simulink model "BaseEngineController_LS"  (Simulink 7.7)
settings: Solver=FixedStepDiscrete  StartTime=0.0  StopTime=10.0  RelTol=1e-3
PreLoadFcn:
  | try, eval([bdroot '_setup']); catch, eval('model_setup', ''); end
InitFcn:
  | try, eval([bdroot '_setup']); catch, eval('model_setup', ''); end
undefined symbols (not defined in the file): ECU555, High, motohawk_build_version, motohawk_trunc_name, motohawk_vardec_config_group, motohawk_vardec_path, True
libraries: MotoHawk_lib x1418, motohawk_control_primitives_lib x183, motohawk_engine_lib x32, simulink x21, motohawk_annotations_lib x9, AutoDoc_lib x8, simulink_extras x4, motohawk_ccp_examples_lib x1, motohawk_control_primitives_motoshare_lib x1
(part 22 of 27)

== system BaseEngineController_LS/Foreground/Control/Controller/Run/MinGovernor/Idle State Determination ==
  Sensors : Inport
  MinGovOutput : Inport  Port=2
  TargetRPM : Inport  Port=3
  Bus Selector1 : BusSelector  OutputSignals=Raw.RPMInst
  Bus Selector2 : BusSelector  OutputSignals=RawProcessed.APPPcnt,RawProcessed.TPS
  Bus Selector3 : BusSelector  OutputSignals=RawProcessed.ETCRequest
  Constant : Constant  Value=true
  Data Type Conversion : DataTypeConversion  OutDataTypeStr=int16
  Determine if RPM is Falling : Subsystem
  IdleStateMachine : Stateflow chart  TreatAsAtomicUnit=on
      settings: RTWSystemCode=Function  RTWFcnNameOpts=Use subsystem name  RTWFileNameOpts=Use function name
  Logical Operator : Logic  OutDataTypeStr=boolean
  Multiport Switch : MultiPortSwitch  DataPortOrder=Zero-based contiguous  Inputs=2  zeroidx=on
  Multiport Switch1 : MultiPortSwitch  DataPortOrder=Zero-based contiguous  Inputs=2  zeroidx=on
  OnIdle State : motohawk_control_primitives_lib/CompareTo  SystemSampleTime=-1  op===  val=2
  Relational Operator : RelationalOperator  Operator=<  ZeroCross=off  InputSameDT=on
  Relational Operator1 : RelationalOperator  Operator=<  ZeroCross=off  InputSameDT=on
  Relational Operator2 : RelationalOperator  ZeroCross=off  InputSameDT=on
  Relational Operator3 : RelationalOperator  Operator=<  ZeroCross=off  InputSameDT=on
  Relational Operator4 : RelationalOperator  Operator=>  OutDataTypeStr=boolean
  Relational Operator5 : RelationalOperator  Operator=>  ZeroCross=off  InputSameDT=on
  Sum : Sum  Inputs=|++  SaturateOnIntegerOverflow=on  InputSameDT=on
  Sum1 : Sum  Inputs=++|  SaturateOnIntegerOverflow=on  InputSameDT=on
  Sum2 : Sum  Inputs=+-|  SaturateOnIntegerOverflow=on  InputSameDT=on
  Time Since Enabled (With Input)1 : motohawk_control_primitives_lib/Time Since Enabled (With Input)1  SystemSampleTime=-1  nam='IdleEnterTimer'  samp_time=.005  init=0  upperlim=16000
  motohawk_calibration1 : MotoHawk_lib/Calibration & Probing Blocks/motohawk_calibration  nam='EnableRPMFalling'  val=1  storage=Calibration  show_more=on  name_source=Use Parameter  data_type=Inherit via back propagation  read_level=1  write_level=1  ovr_cals=on  view_as=Number  enum_struct={'Disabled', 'Enabled'}  vector_style=Wide Row  use_help_units=on  help='If disabled, Min Gov will enable immediately after cranking without waiting for falling RPM.'  units='bool'  use_header_enum=off  row_header_enum={}  col_header_enum={}  use_min_max=on  min_val=0  max_val=1  use_precision=off  precision=''  gain=1  offset=0  exp=1  use_mototune_group=on  mototune_group=motohawk_vardec_path(gcb)
  motohawk_calibration2 : MotoHawk_lib/Calibration & Probing Blocks/motohawk_calibration  nam='MinGovEntryAirTimeThresh'  val=10  storage=Calibration  show_more=on  name_source=Use Parameter  data_type=Inherit from 'Default Value'  read_level=1  write_level=1  ovr_cals=on  view_as=Number  enum_struct={'Disabled', 'Enabled'}  vector_style=Wide Row  use_help_units=on  help='If entry AirPcnt condition is satisfied, but RPM is high, Min Gov will enable if this time is exceeded.'  units='s'  use_header_enum=off  row_header_enum={}  col_header_enum={}  use_min_max=on  min_val=-inf  max_val=inf  use_precision=off  precision=''  gain=1  offset=0  exp=1  use_mototune_group=on  mototune_group=motohawk_vardec_path(gcb)
  motohawk_calibration3 : MotoHawk_lib/Calibration & Probing Blocks/motohawk_calibration  nam='MinGovAirPcntHyst'  val=0.5  storage=Calibration  show_more=on  name_source=Use Parameter  data_type=Inherit from 'Default Value'  read_level=1  write_level=1  ovr_cals=on  view_as=Number  enum_struct={'Disabled', 'Enabled'}  vector_style=Wide Row  use_help_units=on  help='Hysteresis around MinGovEntryAirPcnt where Min Gov will disable.'  units='%'  use_header_enum=off  row_header_enum={}  col_header_enum={}  use_min_max=on  min_val=-inf  max_val=inf  use_precision=off  precision=''  gain=1  offset=0  exp=1  use_mototune_group=on  mototune_group=motohawk_vardec_path(gcb)
  motohawk_calibration4 : MotoHawk_lib/Calibration & Probing Blocks/motohawk_calibration  nam='InGearMinGovEntryRPMDelta'  val=75  storage=Calibration  show_more=on  name_source=Use Parameter  data_type=int16  read_level=1  write_level=1  ovr_cals=on  view_as=Number  enum_struct={'Disabled', 'Enabled'}  vector_style=Wide Row  use_help_units=on  help='RPM above setpoint where Min Gov will enable when RPM is falling into idle.'  units='RPM'  use_header_enum=off  row_header_enum={}  col_header_enum={}  use_min_max=on  min_val=-inf  max_val=inf  use_precision=off  precision=''  gain=1  offset=0  exp=1  use_mototune_group=on  mototune_group=motohawk_vardec_path(gcb)
  motohawk_calibration5 : MotoHawk_lib/Calibration & Probing Blocks/motohawk_calibration  nam='MinGovEntryAirPcnt'  val=3  storage=Calibration  show_more=on  name_source=Use Parameter  data_type=Inherit from 'Default Value'  read_level=1  write_level=1  ovr_cals=on  view_as=Number  enum_struct={'Disabled', 'Enabled'}  vector_style=Wide Row  use_help_units=on  help='Percent air (TPS or APP) position where below which Min Gov will enable.'  units='%'  use_header_enum=off  row_header_enum={}  col_header_enum={}  use_min_max=on  min_val=-inf  max_val=inf  use_precision=off  precision=''  gain=1  offset=0  exp=1  use_mototune_group=on  mototune_group=motohawk_vardec_path(gcb)
  motohawk_calibration6 : MotoHawk_lib/Calibration & Probing Blocks/motohawk_calibration  nam='StallSaverDeltaRPM'  val=10  storage=Calibration  show_more=on  name_source=Use Parameter  data_type=int16  read_level=1  write_level=1  ovr_cals=on  view_as=Number  enum_struct={'Disabled', 'Enabled'}  vector_style=Wide Row  use_help_units=on  help='RPM delta below setpoint where Min Gov will enable to prevent engine stalls.'  units='RPM'  use_header_enum=off  row_header_enum={}  col_header_enum={}  use_min_max=on  min_val=-inf  max_val=inf  use_precision=on  precision=''  gain=1  offset=0  exp=1  use_mototune_group=on  mototune_group=motohawk_vardec_path(gcb)
  motohawk_data_read1 : MotoHawk_lib/Data Storage Blocks/motohawk_data_read  source=Lookup By Name  structure=Scalar  operation=Read scalar from location by index  sz_vec=4  sz_row=2  sz_col=3  typ=boolean  nam='AirControlSource'  checkNull=on  struct_inst_name='Struct1'  struct_nam='MyStruct'
  motohawk_probe : MotoHawk_lib/Calibration & Probing Blocks/motohawk_probe  nam='RPMCtrlMode'  show_more=on  name_source=Use Parameter  read_level=1  view_as=Number  enum_struct={'Disabled', 'Enabled'}  vector_style=Wide Row  use_help_units=on  help=''  units=''  use_header_enum=off  row_header_enum={}  col_header_enum={}  use_precision=on  precision=''  gain=1  offset=0  exp=1  use_mototune_group=on  mototune_group=motohawk_vardec_path(gcb)
  motohawk_probe1 : MotoHawk_lib/Calibration & Probing Blocks/motohawk_probe  nam='IdleState'  show_more=on  name_source=Use Parameter  read_level=1  view_as=Enumeration  enum_struct={'Unknown', 'Flaring', 'OnIdle', 'OffIdle'}  vector_style=Wide Row  use_help_units=on  help='The idle governor may be one of: Flaring, OnIdle, OffIdle'  units=''  use_header_enum=off  row_header_enum={}  col_header_enum={}  use_precision=off  precision=''  gain=1  offset=0  exp=1  use_mototune_group=on  mototune_group=motohawk_vardec_path(gcb)
  OnIdle : Outport
  wires:
  Relational Operator3/1 -> IdleStateMachine/4(RPMLow)
  Sum2/1 -> Relational Operator3/2
  motohawk_calibration6/1 -> Sum2/2
  Relational Operator1/1 -> Time Since Enabled (With Input)1/1, IdleStateMachine/5(ThrCmdLow)
  Relational Operator/1 -> IdleStateMachine/3(RPMInRange)
  OnIdle State/1 -> OnIdle/1, motohawk_probe/1
  IdleStateMachine/1(IdleState) -> OnIdle State/1, motohawk_probe1/1
  motohawk_calibration5/1 -> Relational Operator1/2, Sum1/1
  Sum/1 -> Relational Operator/2
  motohawk_calibration4/1 -> Sum/1
  TargetRPM/1 -> Sum2/1, Sum/2
  Determine if RPM is Falling/1(RPM Falling) -> IdleStateMachine/2(RPMFalling)
  Sensors/1 -> Bus Selector1/1, Bus Selector2/1, Bus Selector3/1
  motohawk_calibration3/1 -> Sum1/2
  Sum1/1 -> Relational Operator2/2
  Bus Selector1/1 -> Determine if RPM is Falling/1(RPM), Data Type Conversion/1  "<RPMInst>"
  MinGovOutput/1 -> Relational Operator4/2
  Logical Operator/1 -> IdleStateMachine/6(ThrCmdHigh)
  Relational Operator2/1 -> Logical Operator/1
  motohawk_calibration1/1 -> IdleStateMachine/1(IdleEnable)
  Time Since Enabled (With Input)1/1 -> Relational Operator5/1
  motohawk_calibration2/1 -> Relational Operator5/2
  Relational Operator5/1 -> IdleStateMachine/7(APPTimeThresh)
  Multiport Switch1/1 -> Relational Operator1/1, Relational Operator2/1
  Bus Selector2/1 -> Multiport Switch1/2  "<APPPcnt>"
  Bus Selector2/2 -> Multiport Switch1/3  "<TPS>"
  motohawk_data_read1/1 -> Multiport Switch1/1, Multiport Switch/1
  Bus Selector3/1 -> Relational Operator4/1  "<ETCRequest>"
  Multiport Switch/1 -> Logical Operator/2
  Relational Operator4/1 -> Multiport Switch/2
  Constant/1 -> Multiport Switch/3
  Data Type Conversion/1 -> Relational Operator3/1, Relational Operator/1

== system BaseEngineController_LS/Foreground/Control/Controller/Run/MinGovernor/MotoringDetection ==
  ActualRPM : Inport
  SetpointRPM : Inport  Port=2
  Data Type Conversion : DataTypeConversion  SaturateOnIntegerOverflow=on  RndMeth=Zero
  Relational Operator1 : RelationalOperator  Operator=>
  Relational Operator2 : RelationalOperator  Operator=>
  Sum : Sum  Inputs=+-  SaturateOnIntegerOverflow=on
  Time Since Enabled (With Input)2 : motohawk_control_primitives_lib/Time Since Enabled (With Input)1  SystemSampleTime=-1  nam='MotoringTimer'  samp_time=.005  init=0  upperlim=16000
  motohawk_calibration1 : MotoHawk_lib/Calibration & Probing Blocks/motohawk_calibration  nam='MotoringDtctTimerLimit'  val=5  storage=Calibration  show_more=on  name_source=Use Parameter  data_type=Inherit from 'Default Value'  read_level=1  write_level=1  ovr_cals=on  view_as=Number  enum_struct={'Disabled', 'Enabled'}  vector_style=Wide Row  use_help_units=on  help='Amount of time engine speed has to be above the min gov. rpm set pt to set motoring flag.'  units='sec'  use_header_enum=off  row_header_enum={}  col_header_enum={}  use_min_max=off  min_val=0  max_val=100  use_precision=off  precision=''  gain=1  offset=0  exp=1  use_mototune_group=on  mototune_group=motohawk_vardec_path(gcb)
  motohawk_calibration3 : MotoHawk_lib/Calibration & Probing Blocks/motohawk_calibration  nam='MotoringDeltaRPMLimit'  val=200  storage=Calibration  show_more=on  name_source=Use Parameter  data_type=int16  read_level=1  write_level=1  ovr_cals=on  view_as=Number  enum_struct={'Disabled', 'Enabled'}  vector_style=Wide Row  use_help_units=on  help='This is the amount RPM must be above the Setpoint RPM to set a Motorin Flag.'  units='RPM'  use_header_enum=off  row_header_enum={}  col_header_enum={}  use_min_max=on  min_val=-inf  max_val=inf  use_precision=off  precision=''  gain=1  offset=0  exp=1  use_mototune_group=on  mototune_group=motohawk_vardec_path(gcb)
  motohawk_probe : MotoHawk_lib/Calibration & Probing Blocks/motohawk_probe  nam='MotoringDetectionTime'  show_more=on  name_source=Use Parameter  read_level=1  view_as=Number  enum_struct={'Disabled', 'Enabled'}  vector_style=Wide Row  use_help_units=off  help=''  units=''  use_header_enum=off  row_header_enum={}  col_header_enum={}  use_precision=off  precision=''  gain=1  offset=0  exp=1  use_mototune_group=on  mototune_group=motohawk_vardec_path(gcb)
  motohawk_probe1 : MotoHawk_lib/Calibration & Probing Blocks/motohawk_probe  nam='MotoringDetectionFlag'  show_more=on  name_source=Use Parameter  read_level=1  view_as=Number  enum_struct={'Disabled', 'Enabled'}  vector_style=Wide Row  use_help_units=off  help=''  units=''  use_header_enum=off  row_header_enum={}  col_header_enum={}  use_precision=off  precision=''  gain=1  offset=0  exp=1  use_mototune_group=on  mototune_group=motohawk_vardec_path(gcb)
  MotoringFlag : Outport
  wires:
  Relational Operator2/1 -> Time Since Enabled (With Input)2/1
  Data Type Conversion/1 -> MotoringFlag/1
  motohawk_calibration3/1 -> Relational Operator2/2
  Sum/1 -> Relational Operator2/1
  SetpointRPM/1 -> Sum/2
  Relational Operator1/1 -> Data Type Conversion/1, motohawk_probe1/1
  ActualRPM/1 -> Sum/1
  motohawk_calibration1/1 -> Relational Operator1/2
  Time Since Enabled (With Input)2/1 -> motohawk_probe/1, Relational Operator1/1

== system BaseEngineController_LS/Foreground/Control/Controller/Run/MinGovernor/Ramp RPM ==
  note: 1st-Order Ramp Down
  note: y[k] = a*x[k] + (1-a)*y[k-1]
  note: where a = t/T
  OnIdle : Inport
  TargetRPM : Inport  Port=2
  RPM : Inport  Port=3
  Constant : Constant  OutDataTypeStr=Inherit: Inherit via back propagation
  Don't allow setpoint to ever drop below the TargetRPM : MinMax  Function=max  Inputs=2  SaturateOnIntegerOverflow=on  InputSameDT=on
  Logical Operator : Logic  Operator=NOT
  Preload lowpass filter with current RPM while not on Idle : Switch  Threshold=0.5  ZeroCross=off  SaturateOnIntegerOverflow=on  InputSameDT=on
  Product1 : Product  Inputs=*/  SaturateOnIntegerOverflow=on  InputSameDT=on  OutDataTypeStr=Inherit: Same as first input
  Product2 : Product  SaturateOnIntegerOverflow=on  InputSameDT=on  OutDataTypeStr=Inherit: Same as first input
  Product3 : Product  SaturateOnIntegerOverflow=on  InputSameDT=on  OutDataTypeStr=Inherit: Same as first input
  Sum : Sum  Inputs=-+|  SaturateOnIntegerOverflow=on
  Sum1 : Sum  SaturateOnIntegerOverflow=on
  Unit Delay : UnitDelay  SampleTime=-1
  motohawk_calibration2 : MotoHawk_lib/Calibration & Probing Blocks/motohawk_calibration  nam='InGearRPMCtrlEntryFiltC'  val=0.1  storage=Calibration  show_more=on  name_source=Use Parameter  data_type=Inherit from 'Default Value'  read_level=1  write_level=1  ovr_cals=on  view_as=Number  enum_struct={'Disabled', 'Enabled'}  vector_style=Wide Row  use_help_units=on  help='Sets decay rate of RPM setpoint from entry RPM.'  units='sec'  use_header_enum=off  row_header_enum={}  col_header_enum={}  use_min_max=on  min_val=.005  max_val=inf  use_precision=off  precision=''  gain=1  offset=0  exp=1  use_mototune_group=on  mototune_group=motohawk_vardec_path(gcb)
  motohawk_delta_time : MotoHawk_lib/Extra Development Blocks/motohawk_delta_time  samp_time=-1  init_val=0  mode=Seconds (double)
  motohawk_probe1 : MotoHawk_lib/Calibration & Probing Blocks/motohawk_probe  nam='MinGovRPMSetPt'  show_more=on  name_source=Use Parameter  read_level=1  view_as=Number  enum_struct={'Disabled', 'Enabled'}  vector_style=Wide Row  use_help_units=on  help=''  units=''  use_header_enum=off  row_header_enum={}  col_header_enum={}  use_precision=on  precision=''  gain=1  offset=0  exp=1  use_mototune_group=on  mototune_group=motohawk_vardec_path(gcb)
  RPMSetPt : Outport
  wires:
  Logical Operator/1 -> Preload lowpass filter with current RPM while not on Idle/2
  Don't allow setpoint to ever drop below the TargetRPM/1 -> RPMSetPt/1, Unit Delay/1, motohawk_probe1/1
  Preload lowpass filter with current RPM while not on Idle/1 -> Don't allow setpoint to ever drop below the TargetRPM/2
  RPM/1 -> Preload lowpass filter with current RPM while not on Idle/1
  TargetRPM/1 -> Don't allow setpoint to ever drop below the TargetRPM/1, Product2/1
  Product1/1 -> Sum/1, Product2/2  "alpha"
  Constant/1 -> Sum/2
  Product2/1 -> Sum1/1
  Product3/1 -> Sum1/2
  Sum/1 -> Product3/1
  Unit Delay/1 -> Product3/2
  motohawk_delta_time/1 -> Product1/1
  motohawk_calibration2/1 -> Product1/2
  Sum1/1 -> Preload lowpass filter with current RPM while not on Idle/3
  OnIdle/1 -> Logical Operator/1

== system BaseEngineController_LS/Foreground/Control/Controller/Run/MinGovernor/Universal PD (Tunable & Scheduled) ==
  Actual : Inport
  SetPoint : Inport  Port=2
  ResetAll : Inport  Port=3
  Constant1 : Constant  Value=0
  PID Gain Select : Subsystem
  Saturation : motohawk_control_primitives_lib/Saturation  SystemSampleTime=-1
  Switch : Switch  Threshold=0.5
  Universal PD : motohawk_control_primitives_lib/Universal PD  Description=|  SystemSampleTime=-1  samp_time=.005
      | /* Name: ErrorGain Unit:mult ClassID:VAR StorageID:FLASH Access:RW4+RW3+NA2+NA1 TypeID:UINT4                   
      |    Gain:0.000000001 Min:0.000000000 Max:4.000000000 Format:10.9 UpdateID:REMOTE Help:"This gain is applied to "
      |    "the error term before it is used to calculate the P, I and D terms." VardecSig:6C */                       
      |                                                                                                                
      | /* Name: ITermLowerLim Unit:0 ClassID:VAR StorageID:FLASH Access:RW4+RW3+NA2+NA1 TypeID:SINT2 Gain:0.1         
      |    Min:-3276.8 Max:3276.7 Format:5.1 UpdateID:REMOTE Help:"Lower limit on the I-term value." VardecSig:6C */   
      |                                                                                                                
      | /* Name: ITermUpperLim ClassID:VAR StorageID:FLASH Access:RW4+RW3+NA2+NA1 TypeID:SINT2 Gain:0.1 Min:-3276.8    
      |    Max:3276.7 Format:5.1 UpdateID:REMOTE Help:"Upper limit on I-term value." VardecSig:6C */                   
      |                                                                                                                
      | /* Name: PIDOutLowerLim ClassID:VAR StorageID:FLASH Access:RW4+RW3+NA2+NA1 TypeID:SINT2 Gain:0.1               
      |    Min:-3276.8 Max:3276.7 Format:5.1 UpdateID:REMOTE Help:"Lower limit on PID output." VardecSig:6C */         
      |                                                                                                                
      | /* Name: PIDOutUpperLim ClassID:VAR StorageID:FLASH Access:RW4+RW3+NA2+NA1 TypeID:SINT2 Gain:0.1               
      |    Min:-3276.8 Max:3276.7 Format:3.1 UpdateID:REMOTE Help:"Upper limit on PID output." VardecSig:6C */
  motohawk_calibration1 : MotoHawk_lib/Calibration & Probing Blocks/motohawk_calibration  nam=[prefix 'PIDOutUpperLimit']  val=3  storage=Calibration  show_more=on  name_source=Use Parameter  data_type=Inherit from 'Default Value'  read_level=1  write_level=1  ovr_cals=on  view_as=Number  enum_struct={'Disabled', 'Enabled'}  vector_style=Wide Row  use_help_units=on  help='Upper limit on spark min governor PID Output.'  units=units  use_header_enum=off  row_header_enum={}  col_header_enum={}  use_min_max=on  min_val=-inf  max_val=inf  use_precision=off  precision=''  gain=1  offset=0  exp=1  use_mototune_group=on  mototune_group=motohawk_vardec_path(gcb)
  motohawk_calibration4 : MotoHawk_lib/Calibration & Probing Blocks/motohawk_calibration  nam=[prefix 'ErrorGain']  val=0.2  storage=Calibration  show_more=on  name_source=Use Parameter  data_type=Inherit from 'Default Value'  read_level=1  write_level=1  ovr_cals=on  view_as=Number  enum_struct={'Disabled', 'Enabled'}  vector_style=Wide Row  use_help_units=on  help='Error gain for the min governor controller. This gain is applied to the RPM error term before it is used to calculate the P, I and D terms.'  units='mult'  use_header_enum=off  row_header_enum={}  col_header_enum={}  use_min_max=on  min_val=-inf  max_val=inf  use_precision=off  precision=''  gain=1  offset=0  exp=1  use_mototune_group=on  mototune_group=motohawk_vardec_path(gcb)
  motohawk_calibration9 : MotoHawk_lib/Calibration & Probing Blocks/motohawk_calibration  nam=[prefix 'PIDOutLowerLimit']  val=-6  storage=Calibration  show_more=on  name_source=Use Parameter  data_type=Inherit from 'Default Value'  read_level=1  write_level=1  ovr_cals=on  view_as=Number  enum_struct={'Disabled', 'Enabled'}  vector_style=Wide Row  use_help_units=on  help='Lower limit on spark min governor PID Output.'  units=units  use_header_enum=off  row_header_enum={}  col_header_enum={}  use_min_max=on  min_val=-inf  max_val=inf  use_precision=off  precision=''  gain=1  offset=0  exp=1  use_mototune_group=on  mototune_group=motohawk_vardec_path(gcb)
  motohawk_prelookup1 : MotoHawk_lib/Lookup Tables/motohawk_prelookup  nam=[prefix 'SpeedError']  breakpoint_data=[-250 -125 -30 30 67 103 140 177 213]  show_more=on  data_type=Inherit from 'Table Data'  storage=Constant  read_level=1  write_level=1  ovr_cals=on  use_help=on  help=''  units=''  use_min_max=off  min_val=-inf  max_val=inf  use_precision=on  precision=''  gain=1  offset=0  exp=1  use_links=off  input_name=''  use_mototune_group=on  mototune_group=motohawk_vardec_path(gcb)
  motohawk_probe1 : MotoHawk_lib/Calibration & Probing Blocks/motohawk_probe  nam=[prefix 'PTerm']  show_more=on  name_source=Use Parameter  read_level=1  view_as=Number  enum_struct={'Disabled', 'Enabled'}  vector_style=Wide Row  use_help_units=on  help='PID Proportional Term'  units=units  use_header_enum=off  row_header_enum={}  col_header_enum={}  use_precision=off  precision=''  gain=1  offset=0  exp=1  use_mototune_group=on  mototune_group=motohawk_vardec_path(gcb)
  motohawk_probe3 : MotoHawk_lib/Calibration & Probing Blocks/motohawk_probe  nam=[prefix 'DTerm']  show_more=on  name_source=Use Parameter  read_level=1  view_as=Number  enum_struct={'Disabled', 'Enabled'}  vector_style=Wide Row  use_help_units=on  help='PID Derivative Term'  units=units  use_header_enum=off  row_header_enum={}  col_header_enum={}  use_precision=off  precision=''  gain=1  offset=0  exp=1  use_mototune_group=on  mototune_group=motohawk_vardec_path(gcb)
  motohawk_probe4 : MotoHawk_lib/Calibration & Probing Blocks/motohawk_probe  nam=[prefix 'Error']  show_more=on  name_source=Use Parameter  read_level=1  view_as=Number  enum_struct={'Disabled', 'Enabled'}  vector_style=Wide Row  use_help_units=on  help='PID Error Term'  units=units  use_header_enum=off  row_header_enum={}  col_header_enum={}  use_precision=off  precision=''  gain=1  offset=0  exp=1  use_mototune_group=on  mototune_group=motohawk_vardec_path(gcb)
  SpkOut : Outport
  wires:
  motohawk_prelookup1/1 -> PID Gain Select/1(ErrorIdx)
  PID Gain Select/2(DGain) -> Universal PD/5
  PID Gain Select/1(PGain) -> Universal PD/4
  motohawk_calibration4/1 -> Universal PD/3
  Universal PD/3 -> motohawk_probe1/1
  Universal PD/1 -> Saturation/1
  Universal PD/4 -> motohawk_probe3/1
  Universal PD/2 -> motohawk_probe4/1, motohawk_prelookup1/1
  Saturation/1 -> Switch/3
  Actual/1 -> Universal PD/1
  SetPoint/1 -> Universal PD/2
  motohawk_calibration1/1 -> Saturation/3
  motohawk_calibration9/1 -> Saturation/2
  Constant1/1 -> Switch/1
  Switch/1 -> SpkOut/1
  ResetAll/1 -> Switch/2

== system BaseEngineController_LS/Foreground/Control/Controller/Run/MinGovernor/Universal PID (Tunable & Scheduled) ==
  Actual : Inport
  SetPoint : Inport  Port=2
  ResetAll : Inport  Port=3
  Constant : Constant  Value=0  OutDataTypeStr=Inherit: Inherit via back propagation
  Constant1 : Constant  Value=0
  PID Gain Select1 : Subsystem
  Saturation : motohawk_control_primitives_lib/Saturation  SystemSampleTime=-1
  Switch : Switch  Threshold=0.5
  Universal PID : motohawk_control_primitives_lib/Universal PID  Description=|  SystemSampleTime=-1  samp_time=.005
      | /* Name: ErrorGain Unit:mult ClassID:VAR StorageID:FLASH Access:RW4+RW3+NA2+NA1 TypeID:UINT4                   
      |    Gain:0.000000001 Min:0.000000000 Max:4.000000000 Format:10.9 UpdateID:REMOTE Help:"This gain is applied to "
      |    "the error term before it is used to calculate the P, I and D terms." VardecSig:6C */                       
      |                                                                                                                
      | /* Name: ITermLowerLim Unit:0 ClassID:VAR StorageID:FLASH Access:RW4+RW3+NA2+NA1 TypeID:SINT2 Gain:0.1         
      |    Min:-3276.8 Max:3276.7 Format:5.1 UpdateID:REMOTE Help:"Lower limit on the I-term value." VardecSig:6C */   
      |                                                                                                                
      | /* Name: ITermUpperLim ClassID:VAR StorageID:FLASH Access:RW4+RW3+NA2+NA1 TypeID:SINT2 Gain:0.1 Min:-3276.8    
      |    Max:3276.7 Format:5.1 UpdateID:REMOTE Help:"Upper limit on I-term value." VardecSig:6C */                   
      |                                                                                                                
      | /* Name: PIDOutLowerLim ClassID:VAR StorageID:FLASH Access:RW4+RW3+NA2+NA1 TypeID:SINT2 Gain:0.1               
      |    Min:-3276.8 Max:3276.7 Format:5.1 UpdateID:REMOTE Help:"Lower limit on PID output." VardecSig:6C */         
      |                                                                                                                
      | /* Name: PIDOutUpperLim ClassID:VAR StorageID:FLASH Access:RW4+RW3+NA2+NA1 TypeID:SINT2 Gain:0.1               
      |    Min:-3276.8 Max:3276.7 Format:3.1 UpdateID:REMOTE Help:"Upper limit on PID output." VardecSig:6C */
  motohawk_calibration2 : MotoHawk_lib/Calibration & Probing Blocks/motohawk_calibration  nam=[prefix 'PIDOutUpperLimit']  val=150  storage=Calibration  show_more=on  name_source=Use Parameter  data_type=Inherit from 'Default Value'  read_level=1  write_level=1  ovr_cals=on  view_as=Number  enum_struct={'Disabled', 'Enabled'}  vector_style=Wide Row  use_help_units=on  help='Upper limit on air min governor PID Output.'  units=units  use_header_enum=off  row_header_enum={}  col_header_enum={}  use_min_max=off  min_val=-inf  max_val=inf  use_precision=off  precision=''  gain=1  offset=0  exp=1  use_mototune_group=on  mototune_group=[group ' | Air PID Config']
  motohawk_calibration5 : MotoHawk_lib/Calibration & Probing Blocks/motohawk_calibration  nam=[prefix 'ErrorGain']  val=0.4  storage=Calibration  show_more=on  name_source=Use Parameter  data_type=Inherit from 'Default Value'  read_level=1  write_level=1  ovr_cals=on  view_as=Number  enum_struct={'Disabled', 'Enabled'}  vector_style=Wide Row  use_help_units=on  help='Error gain for the min governor controller. This gain is applied to the RPM error term before it is used to calculate the P, I and D terms.'  units='mult'  use_header_enum=off  row_header_enum={}  col_header_enum={}  use_min_max=on  min_val=-inf  max_val=inf  use_precision=off  precision=''  gain=1  offset=0  exp=1  use_mototune_group=on  mototune_group=[group ' | Air PID Config']
  motohawk_calibration7 : MotoHawk_lib/Calibration & Probing Blocks/motohawk_calibration  nam=[prefix 'ITermLowerLimit']  val=-3  storage=Calibration  show_more=on  name_source=Use Parameter  data_type=Inherit from 'Default Value'  read_level=1  write_level=1  ovr_cals=on  view_as=Number  enum_struct={'Disabled', 'Enabled'}  vector_style=Wide Row  use_help_units=on  help='Lower limit on Air Min Governor I-term value.'  units=units  use_header_enum=off  row_header_enum={}  col_header_enum={}  use_min_max=on  min_val=-inf  max_val=inf  use_precision=off  precision=''  gain=1  offset=0  exp=1  use_mototune_group=on  mototune_group=[group ' | Air PID Config']
  motohawk_calibration8 : MotoHawk_lib/Calibration & Probing Blocks/motohawk_calibration  nam=[prefix 'ITermUpperLimit']  val=55  storage=Calibration  show_more=on  name_source=Use Parameter  data_type=Inherit from 'Default Value'  read_level=1  write_level=1  ovr_cals=on  view_as=Number  enum_struct={'Disabled', 'Enabled'}  vector_style=Wide Row  use_help_units=on  help='Upper limit on Air Min Governor I-term value.'  units=units  use_header_enum=off  row_header_enum={}  col_header_enum={}  use_min_max=on  min_val=-inf  max_val=inf  use_precision=off  precision=''  gain=1  offset=0  exp=1  use_mototune_group=on  mototune_group=[group ' | Air PID Config']
  motohawk_calibration9 : MotoHawk_lib/Calibration & Probing Blocks/motohawk_calibration  nam=[prefix 'PIDOutLowerLimit']  val=-10  storage=Calibration  show_more=on  name_source=Use Parameter  data_type=Inherit from 'Default Value'  read_level=1  write_level=1  ovr_cals=on  view_as=Number  enum_struct={'Disabled', 'Enabled'}  vector_style=Wide Row  use_help_units=on  help='Lower limit on air min governor PID Output.'  units=units  use_header_enum=off  row_header_enum={}  col_header_enum={}  use_min_max=on  min_val=-inf  max_val=inf  use_precision=off  precision=''  gain=1  offset=0  exp=1  use_mototune_group=on  mototune_group=[group ' | Air PID Config']
  motohawk_prelookup1 : MotoHawk_lib/Lookup Tables/motohawk_prelookup  nam=[prefix 'SpeedError']  breakpoint_data=[-200 -90 -30 0 50 103 140 177 213]  show_more=on  data_type=Inherit from 'Table Data'  storage=Constant  read_level=1  write_level=1  ovr_cals=on  use_help=on  help=''  units=''  use_min_max=off  min_val=-inf  max_val=inf  use_precision=off  precision=''  gain=1  offset=0  exp=1  use_links=off  input_name=''  use_mototune_group=on  mototune_group=motohawk_vardec_path(gcb)
  motohawk_probe1 : MotoHawk_lib/Calibration & Probing Blocks/motohawk_probe  nam=[prefix 'PTerm']  show_more=on  name_source=Use Parameter  read_level=1  view_as=Number  enum_struct={'Disabled', 'Enabled'}  vector_style=Wide Row  use_help_units=on  help='Air min governor P term'  units=''  use_header_enum=off  row_header_enum={}  col_header_enum={}  use_precision=on  precision=''  gain=1  offset=0  exp=1  use_mototune_group=on  mototune_group=motohawk_vardec_path(gcb)
  motohawk_probe2 : MotoHawk_lib/Calibration & Probing Blocks/motohawk_probe  nam=[prefix 'ITerm']  show_more=on  name_source=Use Parameter  read_level=1  view_as=Number  enum_struct={'Disabled', 'Enabled'}  vector_style=Wide Row  use_help_units=on  help='Air min governor I term'  units=''  use_header_enum=off  row_header_enum={}  col_header_enum={}  use_precision=on  precision=''  gain=1  offset=0  exp=1  use_mototune_group=on  mototune_group=motohawk_vardec_path(gcb)
  motohawk_probe3 : MotoHawk_lib/Calibration & Probing Blocks/motohawk_probe  nam=[prefix 'DTerm']  show_more=on  name_source=Use Parameter  read_level=1  view_as=Number  enum_struct={'Disabled', 'Enabled'}  vector_style=Wide Row  use_help_units=on  help='Air min governor D term'  units=''  use_header_enum=off  row_header_enum={}  col_header_enum={}  use_precision=on  precision=''  gain=1  offset=0  exp=1  use_mototune_group=on  mototune_group=motohawk_vardec_path(gcb)
  motohawk_probe6 : MotoHawk_lib/Calibration & Probing Blocks/motohawk_probe  nam=[prefix 'Error']  show_more=on  name_source=Use Parameter  read_level=1  view_as=Number  enum_struct={'Disabled', 'Enabled'}  vector_style=Wide Row  use_help_units=on  help='Air min governor P term'  units=''  use_header_enum=off  row_header_enum={}  col_header_enum={}  use_precision=on  precision=''  gain=1  offset=0  exp=1  use_mototune_group=on  mototune_group=motohawk_vardec_path(gcb)
  MinGovOut : Outport
  MinGovITerm : Outport  Port=2
  wires:
  motohawk_prelookup1/1 -> PID Gain Select1/1(ErrorIdx)
  PID Gain Select1/3(DGain) -> Universal PID/6
  PID Gain Select1/1(PGain) -> Universal PID/4
  motohawk_calibration5/1 -> Universal PID/3
  Universal PID/1 -> Saturation/1
  Universal PID/5 -> motohawk_probe3/1
  Actual/1 -> Universal PID/1
  SetPoint/1 -> Universal PID/2
  PID Gain Select1/2(IGain) -> Universal PID/5
  Universal PID/2 -> motohawk_prelookup1/1, motohawk_probe6/1
  Universal PID/3 -> motohawk_probe1/1
  Universal PID/4 -> motohawk_probe2/1, MinGovITerm/1
  ResetAll/1 -> Universal PID/10, Switch/2
  Constant/1 -> Universal PID/7
  motohawk_calibration7/1 -> Universal PID/8
  motohawk_calibration8/1 -> Universal PID/9
  motohawk_calibration2/1 -> Saturation/3
  motohawk_calibration9/1 -> Saturation/2
  Constant1/1 -> Switch/1
  Saturation/1 -> Switch/3
  Switch/1 -> MinGovOut/1

== system BaseEngineController_LS/Foreground/Control/Controller/Run/O2 Control/Map O2 Sensors to V8 Cylinders ==
  O2FuelMultA : Inport
  O2FuelMultB : Inport  Port=2
  Multiport Switch{,1..7} (8 alike) : MultiPortSwitch  DataPortOrder=Zero-based contiguous  Inputs=2  zeroidx=on  InputSameDT=on
  Mux : Mux  Inputs=8
  Mux1 : Mux  Inputs=8
  motohawk_calibration : MotoHawk_lib/Calibration & Probing Blocks/motohawk_calibration  nam='O2Cyl1Select'  val=0  storage=Calibration  show_more=on  name_source=Use Parameter  data_type=boolean  read_level=1  write_level=1  ovr_cals=on  view_as=Enumeration  enum_struct={'O2A', 'O2B'}  vector_style=Wide Row  use_help_units=on  help='Select the O2 sensor mapped to cylinder 1'  units=''  use_header_enum=off  row_header_enum={}  col_header_enum={}  use_min_max=off  min_val=-inf  max_val=inf  use_precision=off  precision=''  gain=1  offset=0  exp=1  use_mototune_group=on  mototune_group=motohawk_vardec_path(gcb)
  motohawk_calibration1 : MotoHawk_lib/Calibration & Probing Blocks/motohawk_calibration  nam='O2Cyl2Select'  val=0  storage=Calibration  show_more=on  name_source=Use Parameter  data_type=boolean  read_level=1  write_level=1  ovr_cals=on  view_as=Enumeration  enum_struct={'O2A', 'O2B'}  vector_style=Wide Row  use_help_units=on  help='Select the O2 sensor mapped to cylinder 2'  units=''  use_header_enum=off  row_header_enum={}  col_header_enum={}  use_min_max=off  min_val=-inf  max_val=inf  use_precision=off  precision=''  gain=1  offset=0  exp=1  use_mototune_group=on  mototune_group=motohawk_vardec_path(gcb)
  motohawk_calibration2 : MotoHawk_lib/Calibration & Probing Blocks/motohawk_calibration  nam='O2Cyl3Select'  val=0  storage=Calibration  show_more=on  name_source=Use Parameter  data_type=boolean  read_level=1  write_level=1  ovr_cals=on  view_as=Enumeration  enum_struct={'O2A', 'O2B'}  vector_style=Wide Row  use_help_units=on  help='Select the O2 sensor mapped to cylinder 3'  units=''  use_header_enum=off  row_header_enum={}  col_header_enum={}  use_min_max=off  min_val=-inf  max_val=inf  use_precision=off  precision=''  gain=1  offset=0  exp=1  use_mototune_group=on  mototune_group=motohawk_vardec_path(gcb)
  motohawk_calibration3 : MotoHawk_lib/Calibration & Probing Blocks/motohawk_calibration  nam='O2Cyl4Select'  val=0  storage=Calibration  show_more=on  name_source=Use Parameter  data_type=boolean  read_level=1  write_level=1  ovr_cals=on  view_as=Enumeration  enum_struct={'O2A', 'O2B'}  vector_style=Wide Row  use_help_units=on  help='Select the O2 sensor mapped to cylinder 4'  units=''  use_header_enum=off  row_header_enum={}  col_header_enum={}  use_min_max=off  min_val=-inf  max_val=inf  use_precision=off  precision=''  gain=1  offset=0  exp=1  use_mototune_group=on  mototune_group=motohawk_vardec_path(gcb)
  motohawk_calibration4 : MotoHawk_lib/Calibration & Probing Blocks/motohawk_calibration  nam='O2Cyl5Select'  val=0  storage=Calibration  show_more=on  name_source=Use Parameter  data_type=boolean  read_level=1  write_level=1  ovr_cals=on  view_as=Enumeration  enum_struct={'O2A', 'O2B'}  vector_style=Wide Row  use_help_units=on  help='Select the O2 sensor mapped to cylinder 5'  units=''  use_header_enum=off  row_header_enum={}  col_header_enum={}  use_min_max=off  min_val=-inf  max_val=inf  use_precision=off  precision=''  gain=1  offset=0  exp=1  use_mototune_group=on  mototune_group=motohawk_vardec_path(gcb)
  motohawk_calibration5 : MotoHawk_lib/Calibration & Probing Blocks/motohawk_calibration  nam='O2Cyl6Select'  val=0  storage=Calibration  show_more=on  name_source=Use Parameter  data_type=boolean  read_level=1  write_level=1  ovr_cals=on  view_as=Enumeration  enum_struct={'O2A', 'O2B'}  vector_style=Wide Row  use_help_units=on  help='Select the O2 sensor mapped to cylinder 6'  units=''  use_header_enum=off  row_header_enum={}  col_header_enum={}  use_min_max=off  min_val=-inf  max_val=inf  use_precision=off  precision=''  gain=1  offset=0  exp=1  use_mototune_group=on  mototune_group=motohawk_vardec_path(gcb)
  motohawk_calibration6 : MotoHawk_lib/Calibration & Probing Blocks/motohawk_calibration  nam='O2Cyl7Select'  val=0  storage=Calibration  show_more=on  name_source=Use Parameter  data_type=boolean  read_level=1  write_level=1  ovr_cals=on  view_as=Enumeration  enum_struct={'O2A', 'O2B'}  vector_style=Wide Row  use_help_units=on  help='Select the O2 sensor mapped to cylinder 7'  units=''  use_header_enum=off  row_header_enum={}  col_header_enum={}  use_min_max=off  min_val=-inf  max_val=inf  use_precision=off  precision=''  gain=1  offset=0  exp=1  use_mototune_group=on  mototune_group=motohawk_vardec_path(gcb)
  motohawk_calibration7 : MotoHawk_lib/Calibration & Probing Blocks/motohawk_calibration  nam='O2Cyl8Select'  val=0  storage=Calibration  show_more=on  name_source=Use Parameter  data_type=boolean  read_level=1  write_level=1  ovr_cals=on  view_as=Enumeration  enum_struct={'O2A', 'O2B'}  vector_style=Wide Row  use_help_units=on  help='Select the O2 sensor mapped to cylinder 8'  units=''  use_header_enum=off  row_header_enum={}  col_header_enum={}  use_min_max=off  min_val=-inf  max_val=inf  use_precision=off  precision=''  gain=1  offset=0  exp=1  use_mototune_group=on  mototune_group=motohawk_vardec_path(gcb)
  O2FuelMult [per-cylinder] : Outport
  BankCylSelectCal : Outport  Port=2
  wires:
  Mux1/1 -> BankCylSelectCal/1
  Mux/1 -> O2FuelMult [per-cylinder]/1
  Multiport Switch7/1 -> Mux/8
  Multiport Switch6/1 -> Mux/7
  Multiport Switch5/1 -> Mux/6
  Multiport Switch4/1 -> Mux/5
  Multiport Switch3/1 -> Mux/4
  Multiport Switch2/1 -> Mux/3
  Multiport Switch1/1 -> Mux/2
  Multiport Switch/1 -> Mux/1
  O2FuelMultB/1 -> Multiport Switch7/3, Multiport Switch6/3, Multiport Switch5/3, Multiport Switch4/3, Multiport Switch3/3, Multiport Switch2/3, Multiport Switch1/3, Multiport Switch/3
  O2FuelMultA/1 -> Multiport Switch7/2, Multiport Switch6/2, Multiport Switch5/2, Multiport Switch4/2, Multiport Switch3/2, Multiport Switch2/2, Multiport Switch1/2, Multiport Switch/2
  motohawk_calibration7/1 -> Mux1/8, Multiport Switch7/1
  motohawk_calibration6/1 -> Mux1/7, Multiport Switch6/1
  motohawk_calibration5/1 -> Mux1/6, Multiport Switch5/1
  motohawk_calibration4/1 -> Mux1/5, Multiport Switch4/1
  motohawk_calibration3/1 -> Mux1/4, Multiport Switch3/1
  motohawk_calibration2/1 -> Mux1/3, Multiport Switch2/1
  motohawk_calibration1/1 -> Mux1/2, Multiport Switch1/1
  motohawk_calibration/1 -> Mux1/1, Multiport Switch/1

== system BaseEngineController_LS/Foreground/Control/Controller/Run/O2 Control/O2 Control State Determination ==
  note: Desired equivalence ratio is within a delta of 1.0 (stoichiometric)
  note: There are no O2 sensor faults
  O2 Sensor Fault : Inport
  SSEngOpr : Inport  Port=2
  ECT_KeyUp_Idx : Inport  Port=3
  TimeSinceRun : Inport  Port=4
  DesEquivRatio : Inport  Port=5
  Constant : Constant  OutDataTypeStr=single
  Constant1 : Constant  Value=true
  Logical Operator : Logic  AllPortsSameDT=off
  Logical Operator2 : Logic  Inputs=6
  Logical Operator3 : Logic  Operator=NOT  Inputs=3
  Relational Operator : RelationalOperator  Operator=<=  ZeroCross=off  InputSameDT=on
  Relational Operator1 : RelationalOperator  ZeroCross=off  InputSameDT=on
  Relational Operator5 : RelationalOperator  ZeroCross=off  InputSameDT=on
  Sum : Sum  Inputs=|++  SaturateOnIntegerOverflow=on
  Sum1 : Sum  Inputs=+-|  SaturateOnIntegerOverflow=on
  motohawk_calibration1 : MotoHawk_lib/Calibration & Probing Blocks/motohawk_calibration  nam='EquivRatioDelta'  val=0.3  storage=Calibration  show_more=on  name_source=Use Parameter  data_type=Inherit from 'Default Value'  read_level=1  write_level=1  ovr_cals=on  view_as=Number  enum_struct={'Disabled', 'Enabled'}  vector_style=Wide Row  use_help_units=on  help='Equivalence ratio has to be with this band of 1 to achieve close loop.'  units='EquivRatio'  use_header_enum=off  row_header_enum={}  col_header_enum={}  use_min_max=off  min_val=-inf  max_val=inf  use_precision=off  precision='5.3'  gain=1  offset=0  exp=1  use_mototune_group=on  mototune_group=motohawk_vardec_path(gcb)
  motohawk_calibration2 : MotoHawk_lib/Calibration & Probing Blocks/motohawk_calibration  nam='O2ControlEnable'  val=0  storage=Calibration  show_more=on  name_source=Use Parameter  data_type=boolean  read_level=1  write_level=1  ovr_cals=on  view_as=Enumeration  enum_struct={'Disabled', 'Enabled'}  vector_style=Wide Row  use_help_units=on  help='Enables O2 control'  units='bool'  use_header_enum=off  row_header_enum={}  col_header_enum={}  use_min_max=off  min_val=-inf  max_val=inf  use_precision=off  precision='5.3'  gain=1  offset=0  exp=1  use_mototune_group=on  mototune_group=motohawk_vardec_path(gcb)
  motohawk_interpolation_1d : MotoHawk_lib/Lookup Tables/motohawk_interpolation_1d  nam='O2StartUpDelay'  table_data=zeros(1,09)  show_more=on  data_type=Inherit from 'Table Data'  storage=NonAdaptive  read_level=1  write_level=1  ovr_cals=on  use_help=on  help='Delay O2 enable until TimeSinceRun is greater than this time.'  units='s'  use_min_max=off  min_val=-inf  max_val=inf  use_precision=off  precision=''  gain=1  offset=0  exp=1  use_links=off  prelookup_block=''  output_name=''  use_mototune_group=on  mototune_group=motohawk_vardec_path(gcb)
  motohawk_probe : MotoHawk_lib/Calibration & Probing Blocks/motohawk_probe  nam='O2CtrlMode'  show_more=on  name_source=Use Parameter  read_level=1  view_as=Enumeration  enum_struct={'Open-Loop', 'Closed-Loop'}  vector_style=Wide Row  use_help_units=off  help=''  units=''  use_header_enum=off  row_header_enum={}  col_header_enum={}  use_precision=off  precision=''  gain=1  offset=0  exp=1  use_mototune_group=on  mototune_group=motohawk_vardec_path(gcb)
  motohawk_probe3 : MotoHawk_lib/Calibration & Probing Blocks/motohawk_probe  nam='O2TimeDelay'  show_more=on  name_source=Use Parameter  read_level=1  view_as=Enumeration  enum_struct={'Disabled', 'Enabled'}  vector_style=Wide Row  use_help_units=off  help=''  units=''  use_header_enum=off  row_header_enum={}  col_header_enum={}  use_precision=off  precision=''  gain=1  offset=0  exp=1  use_mototune_group=on  mototune_group=motohawk_vardec_path(gcb)
  motohawk_probe5 : MotoHawk_lib/Calibration & Probing Blocks/motohawk_probe  nam='EnginSteadyState'  show_more=on  name_source=Use Parameter  read_level=1  view_as=Enumeration  enum_struct={'Disabled', 'Enabled'}  vector_style=Wide Row  use_help_units=off  help=''  units=''  use_header_enum=off  row_header_enum={}  col_header_enum={}  use_precision=off  precision=''  gain=1  offset=0  exp=1  use_mototune_group=on  mototune_group=motohawk_vardec_path(gcb)
  motohawk_probe6 : MotoHawk_lib/Calibration & Probing Blocks/motohawk_probe  nam='DesEquivInRange'  show_more=on  name_source=Use Parameter  read_level=1  view_as=Enumeration  enum_struct={'Disabled', 'Enabled'}  vector_style=Wide Row  use_help_units=off  help=''  units=''  use_header_enum=off  row_header_enum={}  col_header_enum={}  use_precision=off  precision=''  gain=1  offset=0  exp=1  use_mototune_group=on  mototune_group=motohawk_vardec_path(gcb)
  motohawk_probe7 : MotoHawk_lib/Calibration & Probing Blocks/motohawk_probe  nam='O2SensorFaults'  show_more=on  name_source=Use Parameter  read_level=1  view_as=Enumeration  enum_struct={'Disabled', 'Enabled'}  vector_style=Wide Row  use_help_units=off  help=''  units=''  use_header_enum=off  row_header_enum={}  col_header_enum={}  use_precision=off  precision=''  gain=1  offset=0  exp=1  use_mototune_group=on  mototune_group=motohawk_vardec_path(gcb)
  motohawk_probe9 : MotoHawk_lib/Calibration & Probing Blocks/motohawk_probe  nam='O2Calibration'  show_more=on  name_source=Use Parameter  read_level=1  view_as=Enumeration  enum_struct={'Disabled', 'Enabled'}  vector_style=Wide Row  use_help_units=off  help=''  units=''  use_header_enum=off  row_header_enum={}  col_header_enum={}  use_precision=off  precision=''  gain=1  offset=0  exp=1  use_mototune_group=on  mototune_group=motohawk_vardec_path(gcb)
  O2Control : Outport
  wires:
  O2 Sensor Fault/1 -> Logical Operator3/1
  Relational Operator1/1 -> Logical Operator/2
  Relational Operator/1 -> Logical Operator/1
  Sum1/1 -> Relational Operator1/2
  Sum/1 -> Relational Operator/2
  DesEquivRatio/1 -> Relational Operator/1, Relational Operator1/1
  Constant/1 -> Sum1/1, Sum/2
  motohawk_calibration1/1 -> Sum1/2, Sum/1
  Logical Operator2/1 -> O2Control/1, motohawk_probe/1
  Logical Operator3/1 -> motohawk_probe7/1, Logical Operator2/3
  Logical Operator/1 -> motohawk_probe6/1, Logical Operator2/2
  SSEngOpr/1 -> motohawk_probe5/1, Logical Operator2/1
  motohawk_calibration2/1 -> motohawk_probe9/1, Logical Operator2/5
  TimeSinceRun/1 -> Relational Operator5/1
  Relational Operator5/1 -> Logical Operator2/6, motohawk_probe3/1
  motohawk_interpolation_1d/1 -> Relational Operator5/2
  ECT_KeyUp_Idx/1 -> motohawk_interpolation_1d/1
  Constant1/1 -> Logical Operator2/4
